simulink model "control"  (R2020b)
settings: Solver=VariableStepAuto  StartTime=0.0  StopTime=300  RelTol=1e-3
settings Model: Creator=mcy  LastModifiedBy=mcy

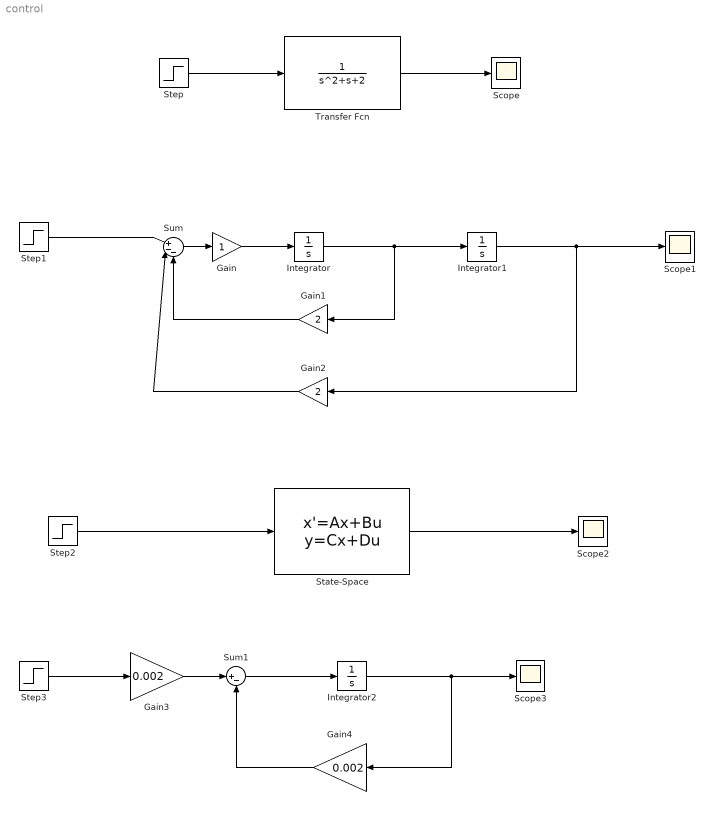
== system control ==
  Gain : Gain
  Gain1 : Gain  Gain=2
  Gain2 : Gain  Gain=2
  Gain3 : Gain  Gain=0.002
  Gain4 : Gain  Gain=0.002
  Integrator : Integrator
  Integrator1 : Integrator
  Integrator2 : Integrator  InitialCondition=300
  Scope{,1..3} (4 alike) : Scope
  State-Space : StateSpace  A=[0 1;-2 -2]  B=[0;1]  C=[1 0]  D=0  InitialCondition=0
  Step : Step  SampleTime=0
  Step1 : Step  SampleTime=0
  Step2 : Step  SampleTime=0
  Step3 : Step  After=326  SampleTime=0
  Sum : Sum  Inputs=|+--
  Sum1 : Sum  Inputs=|+-
  Transfer Fcn : TransferFcn  Denominator=[1 1 2]
  wires:
  Step/1 -> Transfer Fcn/1
  Transfer Fcn/1 -> Scope/1
  Step1/1 -> Sum/1
  Sum/1 -> Gain/1
  Gain/1 -> Integrator/1
  Integrator/1 -> Gain1/1, Integrator1/1
  Gain1/1 -> Sum/3
  Integrator1/1 -> Gain2/1, Scope1/1
  Gain2/1 -> Sum/2
  Step2/1 -> State-Space/1
  State-Space/1 -> Scope2/1
  Integrator2/1 -> Scope3/1, Gain4/1
  Gain4/1 -> Sum1/2
  Step3/1 -> Gain3/1
  Gain3/1 -> Sum1/1
  Sum1/1 -> Integrator2/1
